simulink model "main_sim"  (R2024b)
settings: Solver=ode4  StartTime=0.0  StopTime=1  FixedStep=dt  RelTol=1e-3
settings Model: Creator=ASCL  LastModifiedBy=ASCL

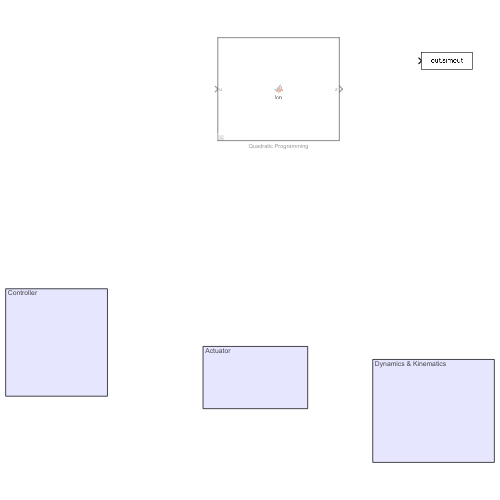
[thumbnail: Simulink's stored preview of the top-level diagram]
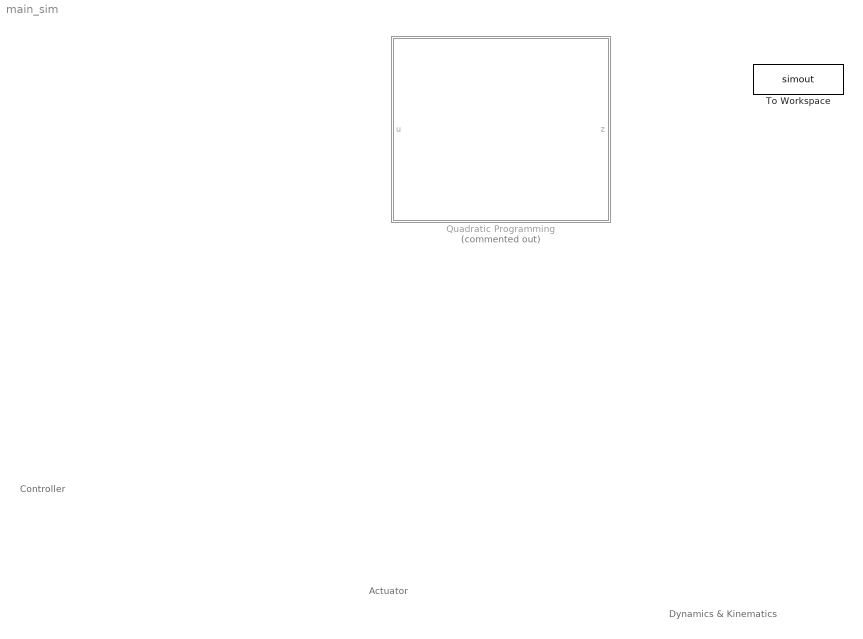
== system main_sim ==
  note: Dynamics & Kinematics
  note: Actuator
  note: Controller
  Quadratic Programming : MATLAB Function  Commented=on  TreatAsAtomicUnit=on
  To Workspace : ToWorkspace  VariableName=simout  SampleTime=-1

== matlab function main_sim/Quadratic Programming ==
  data: u input; z output
function z = fcn(u)
% 입력
% 출력











Aeq = [-P.Cw, P.CT, -eye(3),  zeros(3);
     zeros(3,4), rho*P.CT, zeros(3),   -eye(3)];
beq = [u(i,:), u_h(i,:)]';

A = [-eye(6), zeros(6,6); eye(6),  zeros(6,6)];
B = [T_w_max*ones(4,1); zeros(2,1);  
    T_w_max*ones(4,1); T_T_max*ones(2,1) ];

% Solve QP
opts  = optimoptions('quadprog','Display','off');
[z,~,exitflag] = quadprog(H,f,A,B,Aeq,beq,[],[],[],opts);
